simulink model "model"  (R2021b)
settings: Solver=VariableStepAuto  StartTime=0.0  StopTime=5  RelTol=1e-3
values from neighbouring files (symbols this model uses):
  A = zeros(12)    [Ex1.m]    (also in Ex2.m; Ex3.m; Ex4.m; Ex5.m)
  Ad = eye(size(A)) + Ts*A    [Ex2.m]    (also in Ex3.m = sysd.A; Ex4.m = sysd.A; Ex5.m = sysd.A; systeem.mat = [1 0 0 0 0 0 0 0 0 0 0 0 ... (144 elements, 12x12)])
  B = zeros(12,4)    [Ex1.m]    (also in Ex2.m; Ex3.m; Ex4.m; Ex5.m)
  Bd = Ts*B    [Ex2.m]    (also in Ex3.m = sysd.B; Ex4.m = sysd.B; Ex5.m = sysd.B; systeem.mat = [0 -5.07773769891e-05 0.00033126933 0 -0.00203109507956 0.01)
  C = zeros(6,12)    [Ex1.m]    (also in Ex2.m; Ex3.m = eye(12); Ex4.m; Ex5.m)
  Cd = C    [Ex2.m]    (also in Ex3.m = sysd.C; Ex4.m = sysd.C; Ex5.m = sysd.C; systeem.mat = [0.22360679775 0 0 0 0 0 0 0 0 0 0 0 ... (144 elements, 12x1)
  D = zeros(6,4)    [Ex1.m]    (also in Ex2.m; Ex3.m = zeros(12,4); Ex4.m; Ex5.m)
  Dd = D    [Ex2.m]    (also in Ex3.m = sysd.D; Ex4.m = sysd.D; Ex5.m = sysd.D; systeem.mat = [0 -5.67708333333e-06 3.7037037037e-05 0 -0.000227083333333 )
settings Model: Creator=ninac  LastModifiedBy=hanne

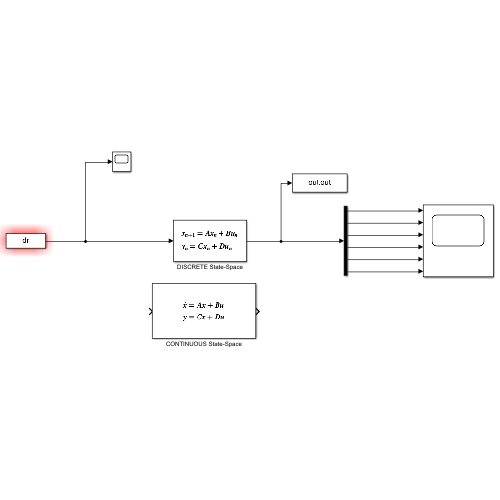
[thumbnail: Simulink's stored preview of the top-level diagram]
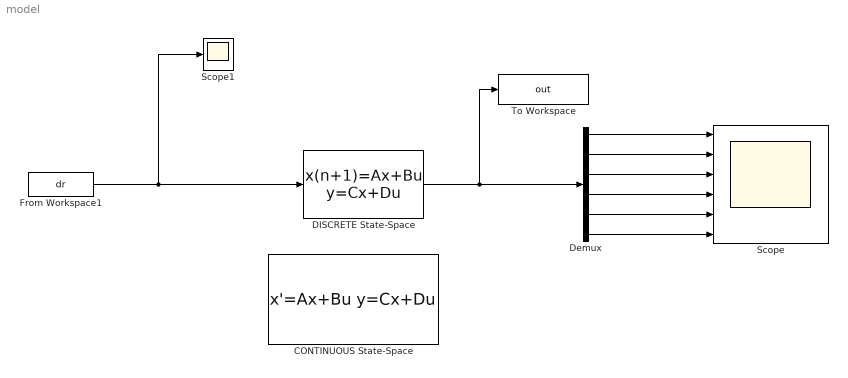
== system model ==
  CONTINUOUS State-Space : StateSpace  A=A  B=B  C=C  D=D  InitialCondition=0
  DISCRETE State-Space : DiscreteStateSpace  A=Ad  B=Bd  C=Cd  D=Dd  SampleTime=0.05
  Demux : Demux  Outputs=6
  From Workspace1 : FromWorkspace  VariableName=dr
  Scope : Scope  NumInputPorts=6
  Scope1 : Scope
  To Workspace : ToWorkspace  VariableName=out  SampleTime=-1
      settings: Save2DSignal=2-D array (concatenate along first dimension)
  wires:
  From Workspace1/1 -> DISCRETE State-Space/1, Scope1/1
  Demux/1 -> Scope/1
  Demux/2 -> Scope/2
  Demux/3 -> Scope/3
  Demux/4 -> Scope/4
  Demux/5 -> Scope/5
  Demux/6 -> Scope/6
  DISCRETE State-Space/1 -> To Workspace/1, Demux/1
